simulink model "MtrCtrl_24V"  (R2023b)
settings: Solver=FixedStepDiscrete  StartTime=0.0  StopTime=1  FixedStep=1e-6  RelTol=1e-3
values from neighbouring files (symbols this model uses):
  B = 0.001889    [MtrCtrl_v01.sldd]    (also in PICal.m = 0.001889; PMSM.m = Simulink.Parameter)
  C_LUT_AngleTable_sng_Null = saveVarsMat.C_LUT_AngleTable_sng_Null    [AngleTable.m]    (also in MtrCtrl_v01.sldd = 0.0015339807878856412 0.0030679615757712823 0.00460194236365; PMSM.m; SinLut.m = sinTable(2,:))
  C_LUT_SinTable_sng_Null = saveVarsMat.C_LUT_SinTable_sng_Null    [AngleTable.m]    (also in MtrCtrl_v01.sldd = 0.0015339801862847655 0.0030679567629659761 0.00460192612044; PMSM.m; SinLut.m = sinTable(1,:))
  C_MATH_OneOverSqrtThree_s32n31_Null = 0.57735026918962584    [MtrCtrl_v01.sldd]    (also in PMSM.m = Simulink.Parameter)
  C_MATH_Pi_u32n30_Null = 3.1415926535897931    [MtrCtrl_v01.sldd]    (also in PMSM.m = Simulink.Parameter)
  C_MATH_SqrtThreeOverThree_s32n31_Null = 0.57735026918962573    [MtrCtrl_v01.sldd]    (also in PMSM.m = Simulink.Parameter)
  C_PMSM_CurQKi_u32n31_null = 0.15707963267949    [MtrCtrl_v01.sldd]    (also in PMSM.m = Simulink.Parameter)
  C_PMSM_CurQKp_u32n31_null = 19.949113350295185    [MtrCtrl_v01.sldd]    (also in PMSM.m = Simulink.Parameter)
  C_PMSM_Flux_u32n32_Vs = 0.192    [MtrCtrl_v01.sldd]    (also in PMSM.m = Simulink.Parameter)
  C_PMSM_Ls_pu = 0.398982267005904    [MtrCtrl_v01.sldd]
  C_PMSM_PolePairs_u8_Null = 4.0    [MtrCtrl_v01.sldd]
  Flux = 0.192    [MtrCtrl_v01.sldd]    (also in PICal.m; PMSM.m)
  IBase_A = 2000.0    [MtrCtrl_v01.sldd]    (also in PICal.m = 300; PMSM.m = Simulink.Parameter)
  J = 0.011    [MtrCtrl_v01.sldd]    (also in PICal.m; PMSM.m)
  K_CCM_MRASEna_bool_Flg = 0.0    [MtrCtrl_v01.sldd]
  K_SVM_DefultDuty_s32n31_Null = 0.25    [MtrCtrl_v01.sldd]    (also in PMSM.m = Simulink.Parameter)
  KCCM_VirPosn_flg = 0.0    [MtrCtrl_v01.sldd]    (also in PMSM.m = Simulink.Parameter)
  KCCM_VoltModeEna_Flg = 0.0    [MtrCtrl_v01.sldd]    (also in PMSM.m = Simulink.Parameter)
  Kis = 114583.3333333333    [MtrCtrl_v01.sldd]    (also in PICal.m = 114583.333333; PMSM.m = 114583.333333)
  KSMO_EnaEst_Flg = 0.0    [MtrCtrl_v01.sldd]    (also in PMSM.m = Simulink.Parameter)
  Kt = 1.1520000000000001    [MtrCtrl_v01.sldd]    (also in PICal.m = 1.152; PMSM.m = 1.152)
  Ld = 80e-6    (= 8e-05)    [FluxweakingGen.m]    (also in IEHB_MAPGenerationtest.m = 6.8e-05; MtrCtrl_v01.sldd = 0.000635
                
                    
             ; PICal.m = 0.000635; PMSM.m = Simulink.Parameter)
  LPF_coefg = 0.01    [MtrCtrl_v01.sldd]    (also in PMSM.m = Simulink.Parameter)
  Lq = 80e-6    (= 8e-05)    [FluxweakingGen.m]    (also in IEHB_MAPGenerationtest.m = 6e-05; MtrCtrl_v01.sldd = 0.000685
                
                    
             ; PICal.m = 0.000635; PMSM.m = Simulink.Parameter)
  Ls = 0.000635    [MtrCtrl_v01.sldd]    (also in PICal.m; PMSM.m)
  OneOverUBase_V = 0.0016666666666666668    [MtrCtrl_v01.sldd]    (also in PMSM.m = Simulink.Parameter)
  Pp = 4.0    [MtrCtrl_v01.sldd]    (also in PICal.m = 4; PMSM.m = Simulink.Parameter)
  Rs = 0.03    [FluxweakingGen.m]    (also in MtrCtrl_v01.sldd = 0.05
                
                    
                 ; PICal.m = 0.05; PMSM.m = Simulink.Parameter)
  SecPerRnd = 0.6    [MtrCtrl_v01.sldd]    (also in PMSM.m = Simulink.Parameter)
  sinTable = zeros(2,TableSize)    [SinLut.m]
  SMOGain_V = 323.31615074619043    [MtrCtrl_v01.sldd]    (also in PMSM.m = Simulink.Parameter)
  Ts = 1.0E-6    [MtrCtrl_v01.sldd]    (also in PICal.m = 0.0001; PMSM.m = Simulink.Parameter)
  TsCtrl = 1.0E-6    [MtrCtrl_v01.sldd]
  UBase_V = 600.0    [MtrCtrl_v01.sldd]    (also in PICal.m = 600; PMSM.m = Simulink.Parameter)
  wmBase_rps = 314.15926535897933    [MtrCtrl_v01.sldd]    (also in PICal.m = 314.159265359; PMSM.m = Simulink.Parameter)
undefined symbols (not defined in the file or in its folder): DiscIntNeverNeededParam, Ion, Lithium
libraries: ee_lib x16, spsVoltageMeasurementLib x14, simulink x11, spsSeriesRLCBranchLib x6, spsMosfetLib x6, nesl_utility x6, slpidlib x5, spsCurrentMeasurementLib x4, spsParallelRLCBranchLib x3, simulink_extras x2, spspowerguiLib x2, eePmsmFwController x1
(part 5 of 5)

== system MtrCtrl_24V/CurLpCtrl/Subsystem10/Subsystem/Cartesian to Polar ==
  In1 : Inport  LockScale=on
  In2 : Inport  Port=2  LockScale=on
  DTC_input_1 : DataTypeConversion  OutDataTypeStr=fixdt('double')  RndMeth=Nearest  SaturateOnIntegerOverflow=off  LockScale=on
  DTC_input_2 : DataTypeConversion  OutDataTypeStr=fixdt('double')  RndMeth=Nearest  SaturateOnIntegerOverflow=off  LockScale=on
  DTC_output_1 : DataTypeConversion  OutDataTypeStr=fixdt(0,32,32)  SaturateOnIntegerOverflow=off  RndMeth=Floor
  DTC_output_2 : DataTypeConversion  OutDataTypeStr=fixdt(1,32,28)  SaturateOnIntegerOverflow=off  RndMeth=Floor
  ReplicaOfSource : simulink_extras/Transformations/Cartesian to Polar
  Out1 : Outport  LockScale=on
  Out2 : Outport  Port=2  LockScale=on
  wires:
  DTC_output_2/1 -> Out2/1
  ReplicaOfSource/1 -> DTC_output_1/1
  DTC_output_1/1 -> Out1/1
  In1/1 -> DTC_input_1/1
  ReplicaOfSource/2 -> DTC_output_2/1
  In2/1 -> DTC_input_2/1
  DTC_input_2/1 -> ReplicaOfSource/2
  DTC_input_1/1 -> ReplicaOfSource/1

== system MtrCtrl_24V/CurLpCtrl/Subsystem10/Subsystem/Polar to Cartesian ==
  In1 : Inport  LockScale=on
  In2 : Inport  Port=2  LockScale=on
  DTC_input_1 : DataTypeConversion  OutDataTypeStr=fixdt('double')  RndMeth=Nearest  SaturateOnIntegerOverflow=off  LockScale=on
  DTC_input_2 : DataTypeConversion  OutDataTypeStr=fixdt('double')  RndMeth=Nearest  SaturateOnIntegerOverflow=off  LockScale=on
  DTC_output_1 : DataTypeConversion  OutDataTypeStr=fixdt(1,32,31)  SaturateOnIntegerOverflow=off  RndMeth=Floor
  DTC_output_2 : DataTypeConversion  OutDataTypeStr=fixdt(1,32,31)  SaturateOnIntegerOverflow=off  RndMeth=Floor
  ReplicaOfSource : simulink_extras/Transformations/Polar to Cartesian
  Out1 : Outport  LockScale=on
  Out2 : Outport  Port=2  LockScale=on
  wires:
  In1/1 -> DTC_input_1/1
  ReplicaOfSource/2 -> DTC_output_2/1
  In2/1 -> DTC_input_2/1
  DTC_input_1/1 -> ReplicaOfSource/1
  ReplicaOfSource/1 -> DTC_output_1/1
  DTC_input_2/1 -> ReplicaOfSource/2
  DTC_output_1/1 -> Out1/1
  DTC_output_2/1 -> Out2/1

== system MtrCtrl_24V/CurLpCtrl/Subsystem10/Subsystem/Subsystem1 ==
  vdq : Inport  OutDataTypeStr=fixdt(1,32,31)
  VphMax : Inport  Port=2  OutDataTypeStr=fixdt(0,32,32)
  Constant : Constant  Value=C_MATH_SqrtThreeOverThree_s32n31_Null
  Math Function : Math  Operator=square  SignedPower=on  OutDataTypeStr=fixdt(0,32,32)
  Product : Product  OutDataTypeStr=Inherit: Inherit via back propagation
  Product1 : Product  Inputs=*/  OutDataTypeStr=fixdt(0,32,31)
  Scope : Scope  NumInputPorts=3
  Sqrt : Sqrt  OutDataTypeStr=fixdt(0,32,32)
  Subsystem : Subsystem
  Sum of Elements : Sum  Inputs=+  OutDataTypeStr=fixdt(0,32,32)
  M : Outport  VectorParamsAs1DForOutWhenUnconnected=off
  wires:
  Sum of Elements/1 -> Sqrt/1
  Subsystem/1(OUT) -> Product1/2, Scope/3
  vdq/1 -> Math Function/1
  Math Function/1 -> Sum of Elements/1
  Product1/1 -> Scope/1, M/1
  Sqrt/1 -> Scope/2, Product1/1
  Product/1 -> Subsystem/1(IN)
  Constant/1 -> Product/2
  VphMax/1 -> Product/1

== system MtrCtrl_24V/CurLpCtrl/Subsystem2/Z_alpha/If Action Subsystem ==
  In1 : Inport  OutDataTypeStr=fixdt(1,32,30)
  Action Port : ActionPort  ActionPortLabel=if(u1 > u2)
  ZalphaOut : Outport
  wires:
  In1/1 -> ZalphaOut/1

== system MtrCtrl_24V/CurLpCtrl/Subsystem2/Z_alpha/If Action Subsystem1 ==
  In1 : Inport  OutDataTypeStr=fixdt(1,32,30)
  Action Port : ActionPort  ActionPortLabel=elseif(u1 < -u2)
  ZalphaOut : Outport
  wires:
  In1/1 -> ZalphaOut/1

== system MtrCtrl_24V/CurLpCtrl/Subsystem2/Z_alpha/If Action Subsystem2 ==
  In1 : Inport  OutDataTypeStr=fixdt(1,32,30)
  Action Port : ActionPort  ActionPortLabel=else
  ZalphaOut : Outport
  wires:
  In1/1 -> ZalphaOut/1

== system MtrCtrl_24V/CurLpCtrl/Subsystem2/Z_alpha1/If Action Subsystem ==
  In1 : Inport  OutDataTypeStr=fixdt(1,32,30)
  Action Port : ActionPort  ActionPortLabel=if(u1 > u2)
  ZalphaOut : Outport
  wires:
  In1/1 -> ZalphaOut/1

== system MtrCtrl_24V/CurLpCtrl/Subsystem2/Z_alpha1/If Action Subsystem1 ==
  In1 : Inport  OutDataTypeStr=fixdt(1,32,30)
  Action Port : ActionPort  ActionPortLabel=elseif(u1 < -u2)
  ZalphaOut : Outport
  wires:
  In1/1 -> ZalphaOut/1

== system MtrCtrl_24V/CurLpCtrl/Subsystem2/Z_alpha1/If Action Subsystem2 ==
  In1 : Inport  OutDataTypeStr=fixdt(1,32,30)
  Action Port : ActionPort  ActionPortLabel=else
  ZalphaOut : Outport
  wires:
  In1/1 -> ZalphaOut/1

== system MtrCtrl_24V/CurLpCtrl/Subsystem10/Subsystem/Subsystem1/Subsystem ==
  IN : Inport  OutDataTypeStr=fixdt(0,32,32)
  Constant2 : Constant  Value=0.1  OutDataTypeStr=fixdt(0,32,32)  SampleTime=-1
  Switch : Switch  Criteria=u2 > Threshold  Threshold=0.1  OutDataTypeStr=fixdt(0,32,32)  SaturateOnIntegerOverflow=off  InputSameDT=off
  OUT : Outport  VectorParamsAs1DForOutWhenUnconnected=off
  wires:
  IN/1 -> Switch/2, Switch/1
  Constant2/1 -> Switch/3
  Switch/1 -> OUT/1

== stateflow chart MtrCtrl_24V/CurLpCtrl/Subsystem5/Chart ==
  (default) -> (junction 2) : {
      | ModAngle = Angle - floor(Angle/(TwoPi))*(TwoPi);
      | Cnt = Angle/(TwoPi);
      | }
  (junction 2) -> (junction 4) [order 1] : [ModAngle <= PiOverTow]
  (junction 2) -> (junction 11) [order 2]
  (junction 4) -> (junction 9) : {
      | SinAngle = ModAngle;
      | SinSign = Pos;
      | CosAngle = PiOverTow - ModAngle;
      | CosSign = Pos;
      | }
  (junction 9) -> (junction 11)
  (junction 11) -> (junction 14)
  (junction 14) -> (junction 16) [order 1] : [ModAngle > PiOverTow && ModAngle <= Pi]
  (junction 14) -> (junction 20) [order 2]
  (junction 16) -> (junction 18) : {
      | SinAngle = Pi - ModAngle;
      | SinSign = Pos;
      | CosAngle = ModAngle - PiOverTow;
      | CosSign = Neg;
      | }
  (junction 18) -> (junction 20)
  (junction 20) -> (junction 23)
  (junction 23) -> (junction 25) [order 1] : [ModAngle > Pi && ModAngle <= PiTimeThreeOverTwo]
  (junction 23) -> (junction 29) [order 2]
  (junction 25) -> (junction 27) : {
      | SinAngle = ModAngle - Pi;
      | SinSign = Neg;
      | CosAngle = PiTimeThreeOverTwo - ModAngle;
      | CosSign = Neg;
      | }
  (junction 27) -> (junction 29)
  (junction 29) -> (junction 40)
  (junction 40) -> (junction 44) [order 1] : [ModAngle > PiTimeThreeOverTwo]
  (junction 40) -> (junction 49) [order 2]
  (junction 44) -> (junction 45) : {
      | SinAngle = Pi + Pi - ModAngle;
      | SinSign = Neg;
      | CosAngle = ModAngle - PiTimeThreeOverTwo;
      | CosSign = Pos;
      | }
  (junction 45) -> (junction 49)
  data: SinAngle output fixdt(0,32,31); PiTimeThreeOverTwo local fixdt(0,32,29) size=1 =pi*3/2; Pi local fixdt(0,32,29) size=1 =pi; PiOverTow local fixdt(0,32,29) size=1 =pi/2; Neg local int8 size=1 =-1; Pos local int8 size=1 =1; SinSign output int8; CosAngle output fixdt(0,32,31); CosSign output int8; ModAngle local fixdt(0,32,29); Angle input fixdt(1,32,26); TwoPi local fixdt(1,32,26) =2*pi; Cnt local fixdt(0,32,29)

== stateflow chart MtrCtrl_24V/CurLpCtrl/SVPWM/Sector/Chart ==
  (default) -> (junction 2) : {
      | Sector = 1;
      | Tx = SqrtThreeOverSix*Udc_pu;
      | Ty = SqrtThreeOverSix*Udc_pu;
      | }
  (junction 2) -> (junction 4) [order 1] : [N == 3]
  (junction 2) -> (junction 6) [order 2]
  (junction 4) -> (junction 19) : {
      | Sector = uint8(3);
      | Tx = Ub;
      | Ty = Ua;
      | }
  (junction 6) -> (junction 22) [order 1] : [N == 1]
  (junction 6) -> (junction 8) [order 2]
  (junction 22) -> (junction 44) : {
      | Sector = uint8(1);
      | Tx = -Ub;
      | Ty = -Uc;
      | }
  (junction 8) -> (junction 39) [order 1] : [N == 5]
  (junction 8) -> (junction 10) [order 2]
  (junction 39) -> (junction 41) : {
      | Sector = uint8(5);
      | Tx = Ua;
      | Ty = Uc;
      | }
  (junction 10) -> (junction 34) [order 1] : [N == 4]
  (junction 10) -> (junction 12) [order 2]
  (junction 34) -> (junction 36) : {
      | Sector = uint8(4);
      | Tx = -Ua;
      | Ty = -Ub;
      | }
  (junction 12) -> (junction 29) [order 1] : [N == 6]
  (junction 12) -> (junction 14) [order 2]
  (junction 29) -> (junction 31) : {
      | Sector = uint8(6);
      | Tx = Uc;
      | Ty = Ub;
      | }
  (junction 14) -> (junction 24) [order 1] : [N == 2]
  (junction 14) -> (junction 15) [order 2]
  (junction 24) -> (junction 26) : {
      | Sector = uint8(2);
      | Tx = -Uc;
      | Ty = -Ua;
      | }
  (junction 26) -> (junction 15)
  (junction 31) -> (junction 26)
  (junction 36) -> (junction 31)
  (junction 41) -> (junction 36)
  (junction 44) -> (junction 41)
  (junction 19) -> (junction 44)
  data: Sector output uint8; Ua input fixdt(1,32,31); Ub input fixdt(1,32,31); Uc input fixdt(1,32,31); Tx output fixdt(1,32,31); Ty output fixdt(1,32,31); N input; Udc_pu local fixdt(0,32,31) =0.0225; SqrtThreeOverSix local fixdt(0,32,31) size=1 [..1] =0.28867513459481288225457439025098

== stateflow chart MtrCtrl_24V/CurLpCtrl/Subsystem2/Subsystem3/Chart ==
  (default) -> (junction 2) : {
      | ModAngle = Angle - floor(Angle/(TwoPi))*(TwoPi);
      | Cnt = Angle/(TwoPi);
      | }
  (junction 2) -> (junction 4) [order 1] : [ModAngle <= PiOverTow]
  (junction 2) -> (junction 11) [order 2]
  (junction 4) -> (junction 9) : {
      | SinAngle = ModAngle;
      | SinSign = Pos;
      | CosAngle = PiOverTow - ModAngle;
      | CosSign = Pos;
      | }
  (junction 9) -> (junction 11)
  (junction 11) -> (junction 14)
  (junction 14) -> (junction 16) [order 1] : [ModAngle > PiOverTow && ModAngle <= Pi]
  (junction 14) -> (junction 20) [order 2]
  (junction 16) -> (junction 18) : {
      | SinAngle = Pi - ModAngle;
      | SinSign = Pos;
      | CosAngle = ModAngle - PiOverTow;
      | CosSign = Neg;
      | }
  (junction 18) -> (junction 20)
  (junction 20) -> (junction 23)
  (junction 23) -> (junction 25) [order 1] : [ModAngle > Pi && ModAngle <= PiTimeThreeOverTwo]
  (junction 23) -> (junction 29) [order 2]
  (junction 25) -> (junction 27) : {
      | SinAngle = ModAngle - Pi;
      | SinSign = Neg;
      | CosAngle = PiTimeThreeOverTwo - ModAngle;
      | CosSign = Neg;
      | }
  (junction 27) -> (junction 29)
  (junction 29) -> (junction 40)
  (junction 40) -> (junction 44) [order 1] : [ModAngle > PiTimeThreeOverTwo]
  (junction 40) -> (junction 49) [order 2]
  (junction 44) -> (junction 45) : {
      | SinAngle = Pi + Pi - ModAngle;
      | SinSign = Neg;
      | CosAngle = ModAngle - PiTimeThreeOverTwo;
      | CosSign = Pos;
      | }
  (junction 45) -> (junction 49)
  data: SinAngle output fixdt(0,32,31); PiTimeThreeOverTwo local fixdt(0,32,29) size=1 =pi*3/2; Pi local fixdt(0,32,29) size=1 =pi; PiOverTow local fixdt(0,32,29) size=1 =pi/2; Neg local int8 size=1 =-1; Pos local int8 size=1 =1; SinSign output int8; CosAngle output fixdt(0,32,31); CosSign output int8; ModAngle local fixdt(0,32,29); Angle input fixdt(1,32,26); TwoPi local fixdt(1,32,26) =2*pi; Cnt local fixdt(0,32,29)

== stateflow chart MtrCtrl_24V/CurLpCtrl/SVPWM/Overmodulation/Chart ==
  (default) -> (junction 2)
  (junction 2) -> (junction 4) [order 1] : [Tx+Ty >= Ts*TwoTimeSqrtThreeOverThree]
  (junction 4) -> (junction 6) [order 1] : [Tx>Ty]
  (junction 2) -> (junction 29) [order 2] : {
      | Tx_o = Tx;
      | Ty_o = Ty;
      | }
  (junction 4) -> (junction 1) [order 2]
  (junction 6) -> (junction 9) : {
      | Tx_o = Ts;
      | Ty_o = 0;
      | }
  (junction 1) -> (junction 12) [order 1] : [Ty > Tx]
  (junction 1) -> (junction 16) [order 2]
  (junction 12) -> (junction 14) : {
      | Tx_o = 0;
      | Ty_o = Ts;
      | }
  (junction 16) -> (junction 18) [order 1] : [Ty > Ts && Ts > Tx]
  (junction 16) -> (junction 25) [order 2] : {
      | m = Ts/(Tx+Ty);
      | Tx_o = Tx * m;
      | Ty_o = Ty * m;
      | }
  (junction 18) -> (junction 20) : {
      | Tx_o = 0;
      | Ty_o = Ts;
      | }
  (junction 25) -> (junction 29)
  (junction 20) -> (junction 25)
  (junction 14) -> (junction 20)
  (junction 9) -> (junction 14)
  data: Tx_o output fixdt(0,32,30); Ts input; Ty input; Ty_o output fixdt(0,32,30); Tx input; m local fixdt(1,32,4) size=1 =1; TwoTimeSqrtThreeOverThree local fixdt(0,32,30) size=1 =1.15470053814351558685302734375
